simulink model "uavsimblockset_test_zagi"  (Simulink 8.0)
settings: Solver=ode45  StartTime=0.0  StopTime=inf  FixedStep=1/100  RelTol=1e-5
libraries: uavsimBlockset_Environment_calmAtmosphere x1, uavsimBlockset_InstrumentPanel x1, uavsimBlockset_ManualLaw x1, aerolibanimutils x1, uavsimBlockset_UAV3DVisualization x1, uavsimBlockset_ZagiUAS x1, uavsimblockset_PilotCommands x1
settings Model: Creator=Jan  LastModifiedBy=j.bolting
settings SolverCC: ZeroCrossAlgorithm=Adaptive

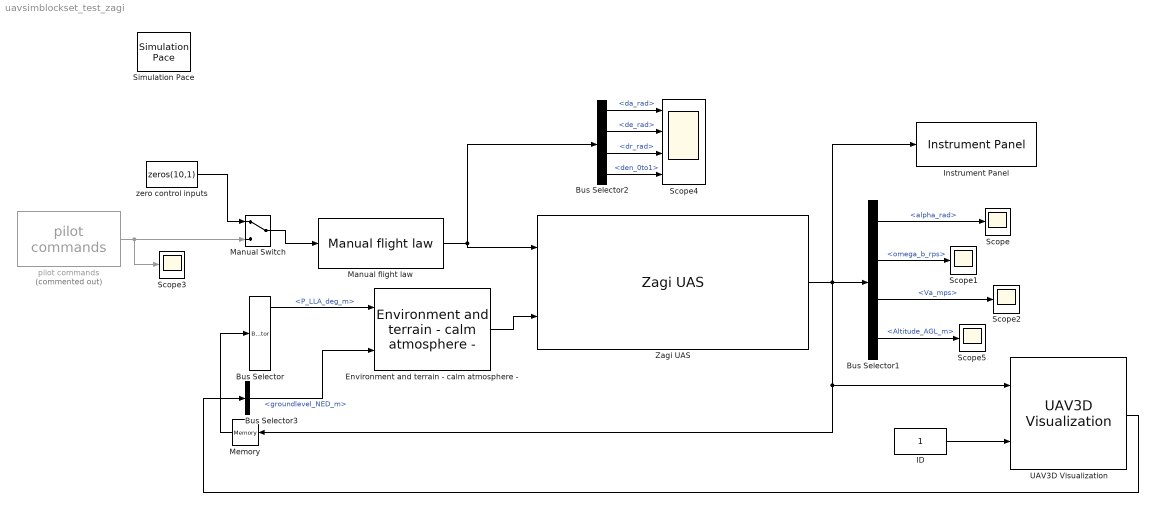
== system uavsimblockset_test_zagi ==
  Bus Selector : BusSelector  OutputSignals=Kinematics.Position.P_LLA_deg_m,Kinematics.Attitude.DCM_be,Aero.Va_mps
  Bus Selector1 : BusSelector  OutputSignals=Aero.alpha_rad,Kinematics.RotationalVelocity.omega_b_rps,Aero.Va_mps,Kinematics.Position.Altitude_AGL_m
  Bus Selector2 : BusSelector  OutputSignals=da_rad,de_rad,dr_rad,den_0to1
  Bus Selector3 : BusSelector  OutputSignals=groundlevel_NED_m
  Environment and terrain - calm atmosphere - : uavsimBlockset_Environment_calmAtmosphere/Environment and terrain - calm atmosphere -  SystemSampleTime=-1
  ID : Constant
  Instrument Panel : uavsimBlockset_InstrumentPanel/Instrument Panel
  Manual Switch : ManualSwitch
  Manual flight law : uavsimBlockset_ManualLaw/Manual flight law  mask_scale_da=deg2rad(-15)  mask_scale_de=deg2rad(30)  mask_scale_dr=deg2rad(0)  mask_scale_den=0  mask_scale_df=deg2rad(0)  mask_utrim=aircraftLibraryData.zagi.u_trim
  Memory : Memory
  Scope{,1..3,5} (5 alike) : Scope
      Scope settings: YMin=0.20206  YMax=0.20229
      Scope2 settings: YMin=11.5  YMax=16.25  SaveName=ScopeData2
      Scope3 settings: SaveName=ScopeData3
      Scope5 settings: TimeRange=10  YMin=-80486  YMax=-80467  SaveName=ScopeData5
  Scope4 : Scope  NumInputPorts=4
      settings: TimeRange=25  YMin=-1~-1~-1~0.475  YMax=1~1~1~0.525  SaveName=ScopeData4
  Simulation Pace : aerolibanimutils/Simulation Pace  SimulationPace=1  SleepMode=MATLAB Thread  OutputPaceError=off  SampleTime=1/30
      settings: AttributesFormatString=%<SimulationPace> sec/sec
  UAV3D Visualization : uavsimBlockset_UAV3DVisualization/UAV3D Visualization
  Zagi UAS : uavsimBlockset_ZagiUAS/Zagi UAS  mask_zagi_phithetapsi0=aircraftLibraryData.zagi.phithetapsi0  mask_zagi_p0_ECEF_lla=aircraftLibraryData.zagi.p0_ECEF_lla_radradm  mask_zagi_pqr0=aircraftLibraryData.zagi.omega0  mask_zagi_uvw0=aircraftLibraryData.zagi.uvw0
      link override Kinematics/LLA to Flat Earth: R=6378137  F=1/298.257223563
  pilot commands : uavsimblockset_PilotCommands/pilot commands  Commented=on
  zero control inputs : Constant  Value=zeros(10,1)
  wires:
  Manual flight law/1 -> Zagi UAS/1, Bus Selector2/1
  Environment and terrain - calm atmosphere -/1 -> Zagi UAS/2
  Bus Selector/1 -> Environment and terrain - calm atmosphere -/1  "<P_LLA_deg_m>"
  Manual Switch/1 -> Manual flight law/1
  pilot commands/1 -> Scope3/1, Manual Switch/2
  zero control inputs/1 -> Manual Switch/1
  Zagi UAS/1 -> Instrument Panel/1, UAV3D Visualization/1, Memory/1, Bus Selector1/1
  Memory/1 -> Bus Selector/1
  Bus Selector1/1 -> Scope/1  "<alpha_rad>"
  Bus Selector1/2 -> Scope1/1  "<omega_b_rps>"
  Bus Selector1/3 -> Scope2/1  "<Va_mps>"
  Bus Selector2/1 -> Scope4/1  "<da_rad>"
  Bus Selector2/2 -> Scope4/2  "<de_rad>"
  Bus Selector2/3 -> Scope4/3  "<dr_rad>"
  Bus Selector2/4 -> Scope4/4  "<den_0to1>"
  ID/1 -> UAV3D Visualization/2
  UAV3D Visualization/1 -> Bus Selector3/1
  Bus Selector1/4 -> Scope5/1  "<Altitude_AGL_m>"
  Bus Selector3/1 -> Environment and terrain - calm atmosphere -/2  "<groundlevel_NED_m>"
